simulink model "homing_ldm_aggiornat"  (R2017a)
settings: Solver=FixedStepAuto  StartTime=0.0  StopTime=inf  FixedStep=1e-3  RelTol=1e-3  EnableMultiTasking=on
libraries: xpcnilib x10, simulink x4
settings Model: SimulationMode=external  Creator=Davide  LastModifiedBy=stefa
settings SolverCC: EnableConcurrentExecution=on  ConcurrentTasks=on  AutoInsertRateTranBlk=on
settings DataIOCC: SaveFormat=StructureWithTime
settings OptimizationCC: BlockReduction=off  OptimizeBlockIOStorage=off  BufferReuse=off  GlobalBufferReuse=off  ExpressionFolding=off  LocalBlockOutputs=off
settings HardwareCC: ProdBitPerPointer=32  ProdBitPerSizeT=32  ProdBitPerPtrDiffT=32  ProdLargestAtomicFloat=None  ProdWordSize=32  ProdLongLongMode=on  ProdHWDeviceType=Generic->32-bit x86 compatible
settings RTWCC: SystemTargetFile=slrt.tlc  TemplateMakefile=slrt_default_tmf  Description=Simulink Real-Time  RTWCompilerOptimization=on
settings SimulinkRealTimeCC: xPCConcurrentTasks=on

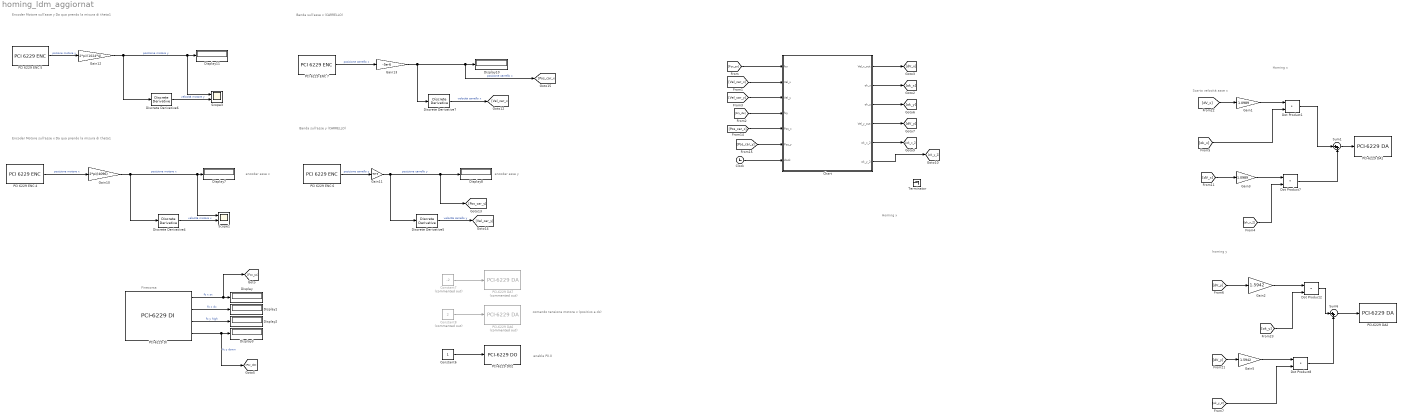
== system homing_ldm_aggiornat ==
  note: Finecorsa
  note: Homing x
  note: Encoder Motore sull'asse y
      | Da qua prendo la misura di theta1
  note: encoder asse y
  note: encoder asse x
  note: Banda sull'asse y (CARRELLO)
  note: comando tensione motore x (positivo a dx)
  note: Encoder Motore sull'asse x
      | Da qua prendo la misura di theta1
  note: enable P0.0
  note: Banda sull'asse x (CARRELLO)
  note: Scarto velocità asse x
  note: Homing x
  note: homing y
  Chart : Stateflow chart  TreatAsAtomicUnit=on
  Clock : Clock
  Constant6 : Constant
  Constant7 : Constant  Commented=on  Value=-2
  Constant8 : Constant  Commented=on  Value=2
  Discrete Derivative{4..7} (4 alike) : simulink/Discrete/Discrete Derivative  gainval=1.0  ICPrevScaledInput=0.0  OutMin=[]  OutMax=[]  OutDataType=fixdt(1, 16)  OutScaling=2^-10  DoSatur=off
  Display{,1..3,7..8,10..11} (8 alike) : Display
  Dot Product{1..2,7..8} (4 alike) : DotProduct  InputSameDT=on  OutDataTypeStr=Inherit: Inherit via internal rule
  Gain1 : Gain  Gain=1.0989
  Gain10 : Gain  Gain=2*pi/(4096)
  Gain11 : Gain  Gain=-5e-6
  Gain12 : Gain  Gain=2*pi/(1024*4)
  Gain13 : Gain  Gain=-5e-6
  Gain2 : Gain  Gain=1.5942
  Gain3 : Gain  Gain=1.0989
  Gain5 : Gain  Gain=1.5942
  PCI 6229 ENC 4 : xpcnilib/Incremental Encoder/PCI 6229 ENC   channel=0  countMode=Quadrature Mode x4  initCount=0  reload=on  indexPhase=A low B low  filter=None  sampleTime=0.001  slot=[4 12]
      settings: SourceProductName=Simulink Real-Time  SourceProductBaseCode=XP
  PCI 6229 ENC 5 : xpcnilib/Incremental Encoder/PCI 6229 ENC   channel=1  countMode=Quadrature Mode x4  initCount=0  reload=on  indexPhase=A low B low  filter=None  sampleTime=0.001  slot=[4 12]
      settings: SourceProductName=Simulink Real-Time  SourceProductBaseCode=XP
  PCI 6229 ENC 6 : xpcnilib/Incremental Encoder/PCI 6229 ENC   channel=0  countMode=Quadrature Mode x4  initCount=0  reload=on  indexPhase=A low B low  filter=None  sampleTime=0.001  slot=[4 15]
      settings: SourceProductName=Simulink Real-Time  SourceProductBaseCode=XP
  PCI 6229 ENC 7 : xpcnilib/Incremental Encoder/PCI 6229 ENC   channel=1  countMode=Quadrature Mode x4  initCount=0  reload=on  indexPhase=A low B low  filter=None  sampleTime=0.001  slot=[4 15]
      settings: SourceProductName=Simulink Real-Time  SourceProductBaseCode=XP
  PCI-6229 DA1 : xpcnilib/D//A/M Series/PCI-6229 DA  channel=[1]  reset=[1]  initValue=[0]  sampletime=0.001  slot=[4 12]
      settings: SourceProductName=Simulink Real-Time  SourceProductBaseCode=XP
  PCI-6229 DA2 : xpcnilib/D//A/M Series/PCI-6229 DA  channel=[1]  reset=[1]  initValue=[0]  sampletime=0.001  slot=[4 15]
      settings: SourceProductName=Simulink Real-Time  SourceProductBaseCode=XP
  PCI-6229 DA6 : xpcnilib/D//A/M Series/PCI-6229 DA  Commented=on  channel=[1]  reset=[1]  initValue=[0]  sampletime=0.001  slot=[4 12]
      settings: SourceProductName=Simulink Real-Time  SourceProductBaseCode=XP
  PCI-6229 DA7 : xpcnilib/D//A/M Series/PCI-6229 DA  Commented=on  channel=[1]  reset=[1]  initValue=[0]  sampletime=0.001  slot=[4 15]
      settings: SourceProductName=Simulink Real-Time  SourceProductBaseCode=XP
  PCI-6229 DI : xpcnilib/Digital Input/M Series/PCI-6229 DI  channel=[4 5 6 7]  sampletime=0.001  slot=[4 12]
      settings: SourceProductName=Simulink Real-Time  SourceProductBaseCode=XP
  PCI-6229 DO2 : xpcnilib/Digital Output/M Series/PCI-6229 DO  channel=[1]  reset=[1]  initValue=[0]  sampletime=0.001  slot=[4 12]
      settings: SourceProductName=Simulink Real-Time  SourceProductBaseCode=XP
  Scope1 : Scope  NumInputPorts=2
  Scope3 : Scope  NumInputPorts=2
  Sum1 : Sum  Inputs=|++
  Sum6 : Sum  Inputs=|++
  Terminator : Terminator
  wires:
  PCI-6229 DI/1 -> [Fcx_sx], Display/1  "fc x sx"
  PCI-6229 DI/2 -> Display1/1  "fc x dx"
  PCI-6229 DI/3 -> Display2/1  "fc y high"
  PCI-6229 DI/4 -> [Fcy_dw], Display3/1  "fc y down"
  [Fcx_sx] -> Chart/1(fcx)
  [Vel_car_x] -> Chart/2(Vel_x)
  Chart/1(Vel_x_out) -> [dV_x]
  [Fcy_dw] -> Chart/4(fcy)
  [Vel_car_y] -> Chart/3(Vel_y)
  Chart/2(ok_x) -> [ok_x]
  Chart/3(ok_y) -> [ok_y]
  Chart/4(Vel_y_out) -> [dV_y]
  [Pos_car_x] -> Chart/5(Pos_x)
  Chart/5(ok_x_2) -> [ok_x_2]
  Chart/6(ok_y_2) -> [ok_y_2]
  [Pos_car_y] -> Chart/6(Pos_y)
  Clock/1 -> Chart/7(clock)
  ? -> Terminator/1  "X"
  Gain13/1 -> Discrete Derivative7/1, [Pos_car_x], Display10/1  "posizione carrello x"
  Constant6/1 -> PCI-6229 DO2/1
  Constant8/1 -> PCI-6229 DA6/1
  Discrete Derivative4/1 -> Scope1/2  "velocità motore x"
  Discrete Derivative6/1 -> Scope3/2  "velocità motore y"
  Constant7/1 -> PCI-6229 DA7/1
  PCI 6229 ENC 5/1 -> Gain12/1  "pozione motore y"
  Discrete Derivative7/1 -> [Vel_car_x]  "velocità carrello x"
  Gain11/1 -> [Pos_car_y], Display8/1, Discrete Derivative5/1  "posizione carrello y"
  Gain10/1 -> Display7/1, Scope1/1, Discrete Derivative4/1  "posizione motore x"
  Discrete Derivative5/1 -> [Vel_car_y]  "velocità carrello y"
  PCI 6229 ENC 4/1 -> Gain10/1  "posizione motore x"
  PCI 6229 ENC 6/1 -> Gain11/1  "posizione carrello y"
  PCI 6229 ENC 7/1 -> Gain13/1  "posizione carrello x"
  Gain12/1 -> Scope3/1, Display11/1, Discrete Derivative6/1  "posizione motore y"
  Dot Product2/1 -> Sum6/1
  [dV_y] -> Gain5/1
  Gain3/1 -> Dot Product7/1
  Dot Product8/1 -> Sum6/2
  Sum6/1 -> PCI-6229 DA2/1
  Sum1/1 -> PCI-6229 DA1/1
  Dot Product1/1 -> Sum1/1
  Gain5/1 -> Dot Product8/1
  Gain2/1 -> Dot Product2/1
  [ok_y_2] -> Dot Product8/2
  [ok_x_2] -> Dot Product7/2
  [dV_x] -> Gain3/1
  [ok_x] -> Dot Product1/2
  Dot Product7/1 -> Sum1/2
  Gain1/1 -> Dot Product1/1
  [dV_y] -> Gain2/1
  [dV_x] -> Gain1/1
  [ok_y] -> Dot Product2/2

== stateflow chart homing_ldm_aggiornat/Chart ==
  state Homing1
    state Homing_x
      entry:
      v_sp_x=-2.1;
      v_sp_y=1.2;
      ok_x=1;
      ok_y=1;
      ok_x_2=0;
      during:
      Vel_x_out = v_sp_x-Vel_x;
      Vel_y_out=v_sp_y-Vel_y;
    note: Inizializzazione asse x
        | Inizializzazione asse y
    state Fine_homing1
      entry:
      ok_y=0;
      ok_x=0;
      bx=Pos_x;
      by=Pos_y;
      v_sp_x=2.1;
      v_sp_y=-1.2;
      ok_x_2=1;
      ok_y_2=1;
      during:
      Vel_x_out=v_sp_x-Vel_x;
      dx=Pos_x-bx
      if (dx>0.5 )
      Vel_x_out=0;
      end
      Vel_y_out=v_sp_y-Vel_y;
      dy=abs(Pos_y-by);
      if (dy>0.5 )
      Vel_y_out=0;
      end
    note: Fine inizializzazione
    note: Porto al centro asse x
        | Porto al centro asse y
    state Fine
      entry:
      ok_y_2=0;
      ok_x_2=0;
      inizio_traiettoria=0;
      during:
      inizio_traiettoria=1;
    (default) -> Homing_x
    Homing_x -> Homing1.Fine_homing1 : [fcx==0 && fcy==0]
    Homing1.Fine_homing1 -> Homing1.Fine : [dx>0.5 && dy>0.5]
  state Homing
    state Fine_homing1
      entry:
      ok_y=0;
      ok_x=0;
      a=Pos_x;
      ok_x_2=1;
      t1=clock;
      %X=0;
      %G_=0;
      %F_=0;
      %f_=0;
      during:
      t=clock-t1;
      %[G_,F_,f_]=Constant_Acceleration_ADIM_par(t,[1/3,1/3,1/3]);
      X_=Evaluate_Trajectory(t);
      Vel_x_out=X_;
      dx=Pos_x-a
    state Posizionamento_y
      entry:
      ok_x_2=0;
      ay=Pos_y;
      v_sp_y=-1.3;
      ok_y_2=1;
      during:
      Vel_y_out=v_sp_y-Vel_y;
      dy=abs(Pos_y-ay);
    state Fine
      entry:
      ok_y_2=0;
      ok_x_2=0;
    (default) -> Homing.Fine_homing1 : [fcy==0]
    Homing.Fine_homing1 -> Posizionamento_y : [dx>0.5]
    Posizionamento_y -> Homing.Fine : [dy>0.5]
  (default) -> Homing1
  Homing1.Fine -> Homing : [inizio_traiettoria==1]
  data: t1 local double; t local double; t function_input; X function_output; fcx input; Vel_x_out output; Vel_x input; ok_x output; ok_y output; Vel_y input; Vel_y_out output; fcy input; Pos_x input; dx local; ok_x_2 output; v_sp_x local; a local; v_sp_y local; ay local; Pos_y input; ok_y_2 output; dy local; clock input; bx local; by local; inizio_traiettoria local
  function X=Evaluate_Trajectory(t):
    | function X=Evaluate_Trajectory(t)
    | % parametri:
    | % t: tempo assolu
    | % h: spostamento richiesto
    | y=0;
    | yp=0;
    | ypp=0;
    | X=0;
    | 
    | h=0.5;
    | h0=0;
    | DT=[1/5 1/3 1/3 0]; %ta di ogni singolo ramo perche' composta
    | 
    | par = [1/3, 2/3];
    | 
    | 
    | DT1 = DT(1);
    | DT2 = DT(2);
    | DT3 = DT(3);
    | DT4 = DT(4);
    | 
    | T0 = 0;
    | T1 = T0 + DT1;
    | T2 = T1 + DT2;
    | T3 = T2 + DT3;
    | T4  = T3 + DT4;                  % Total time
    | 
    | if t >= T0 && t <= T1            % Interval N°1 
    |    td = DT1; %tempo di azionamento
    |    x = (t - T0)/td; %tempo adimensionale
    |    
    |    [G,F,f] = Constant_Acceleration_ADIM_par(x,par);
    |    y = h0 + G*h;
    |    yp = F * h/td;
    |    ypp = f * h/td^2;
    | end
    | 
    | if t > T1 && t <= T2             % Interval N°2 
    |    y = h0 + h;
    |    yp = 0;
    |    ypp = 0;
    | end
    | 
    | if t > T2 && t <= T3             % Interval N°3
    |    td = DT3;
    |    x = (t - T2)/td;
    |    
    |    [G,F,f] = Constant_Acceleration_ADIM_par(x,par);
    | 
    |    y = (h0 + h) - G*h;
    |    yp =  - (F * h/td);
    |    ypp = - (f * h/td^2);
    | end
    | 
    | if t > T3               % Interval N°4    
    |    y = h0;
    |    yp = 0;
    |    ypp = 0;  
    | end
    | Y = [y,yp,ypp];
    | X=yp;%pos, vel, acc
